simulink model "control2_feedback_linearization"  (R2023b)
settings: Solver=VariableStepAuto  StartTime=0.0  StopTime=20  RelTol=1e-3
values from neighbouring files (symbols this model uses):
  d = obs_r+threshold    (= 0.3)    [main.m]
  initial_position = [0,r]    [main.m]
  obs_r = 0.1    [main.m]
  obs_x = [20]    [main.m]
  obs_y = [20]    [main.m]
  parking_position = [0,0]    [main.m]
  r = 1    [main.m]
  T = 2*pi    (= 6.28318530718)    [main.m]
  t_values = 0:dt:T*1.1    [main.m]
  threshold = 0.2    [main.m]
undefined symbols (not defined in the file or in its folder): params
(part 3 of 3)

== matlab function control2_feedback_linearization/One circle detection/one circle detection ==
  data: t input; x input; regulation_flag output; y input; initial_position input; regulation_flag_previous input; constant input
function regulation_flag  = fcn( t, x,y,initial_position, regulation_flag_previous, constant)
if(regulation_flag_previous==0)
    if (abs(initial_position(1)- x)<0.001 && abs(initial_position(2)-y)<0.001 &&(t>constant))
        regulation_flag=1;
    else 
        regulation_flag=0;
    end
else
    regulation_flag =1;
end

== matlab function control2_feedback_linearization/Trajectory generator/Trajectory generator and obstacle detection3/Subsystem1/Whole trajectory calculation + flatness ==
  data: r input; trajectory_x output; t_values input; T input; trajectory_y output; v_d_array output; omega_d_array output; theta_d_array output; recalculate output; recalculate_obs input; d input; blending input; theta11 input; xd input; yd input; recalculate_obs1 output; old_trajectory_x input; old_trajectory_y input
function [trajectory_x, trajectory_y, v_d_array, omega_d_array, theta_d_array, recalculate,recalculate_obs1]  = fcn( r, t_values,T, recalculate_obs,d, blending, theta11, xd, yd,old_trajectory_x, old_trajectory_y)
    if(~recalculate_obs)
        trajectory_x = zeros(length(t_values), 1);
        trajectory_y = ones(length(t_values), 1);
        % Triangle parameters
        W = 4;  % Base width
        H = 3;  % Height
        x0 = 0;  % Starting x-coordinate
        y0 = 1;  % Starting y-coordinate

        for i = 1:length(t_values)
            t = t_values(i);
            
            if t < T/3
                % Move up diagonally (first leg)
                trajectory_x(i) = x0 + (W/2) * (t / (T/3));
                trajectory_y(i) = y0 + H * (t / (T/3));
                
            elseif t < 2*T/3
                % Move down diagonally (second leg)
                trajectory_x(i) = x0 + (W/2) + (W/2) * ((t - T/3) / (T/3));
                trajectory_y(i) = y0 + H - H * ((t - T/3) / (T/3));
                
            elseif t<T
                % Move horizontally back to start (third leg)
                trajectory_x(i) = x0 + W - W * ((t - 2*T/3) / (T/3));
                trajectory_y(i) = y0;
            else
                trajectory_x(i) = x0;
                trajectory_y(i) = y0;
            end
        end

    else
        % Obstacle was detected: in the point x, y with angle theta
        W = 4;  % Base width
        H = 3;  % Height
        x0 = 0;  % Starting x-coordinate
        y0 = 1;  % Starting y-coordinate
        center_trajectory = [x0+W/2, y0+H/2];
        % Loading previous version of the trajectory 
        % to avoid additional and useless computations of
        % previous desired path
        trajectory_x = old_trajectory_x;
        trajectory_y = old_trajectory_y;
        x1 = xd;
        y1 = yd;
        points = [trajectory_x,trajectory_y];
        [~, start_idx] = min(vecnorm(points - [x1,y1], 2, 2));

        theta1 = -theta11+pi/2;  % Adjusting the angle to get the anglefrom vertical axis (theta11 is wrt horisontal axis)

        % Estimate the obstacle location
        theta_range = linspace(theta1 - pi/4, theta1 + pi/4, 300);
        x_arc = x1 + d * sin(theta_range);
        y_arc = y1 + d * cos(theta_range);



        % Loop through the trajectory points to check for intersections

        obs_x = x1;
        obs_y = y1;
        obs_idx = start_idx;
        for i = start_idx:length(trajectory_x) - 1
            x_traj_seg = [trajectory_x(i), trajectory_x(i + 1)];
            y_traj_seg = [trajectory_y(i), trajectory_y(i + 1)];
            
            for j = 1:length(x_arc) - 1
                x_arc_seg = [x_arc(j), x_arc(j + 1)];
                y_arc_seg = [y_arc(j), y_arc(j + 1)];
                
                % Check if the two segments intersect
                [intersects, ix, iy] = segmentIntersection(x_traj_seg, y_traj_seg, x_arc_seg, y_arc_seg);
        
                if intersects
                    % Intersection found, assign coordinates
                    obs_x = ix;
                    obs_y = iy;
                    obs_idx = i;
                    break; % Exit the loop once intersection is found
                end
             end
            if obs_x ~= x1
                break; 
            end
        end

        % -- > Finding the point where the obstacle avoidance trajectory should 
        % be finished, point from which the robot should continue on
        % the regular trajectory.Creating a circle of radius d, with the 
        % center in [center_obs_x, center_obs_y].
        % After that, finding an intersection of that circle with the 
        % previous trajectory.
    
        theta_values = linspace(0, 2*pi, 500);
        x_circle = obs_x + d * cos(theta_values);
        y_circle = obs_y + d * sin(theta_values);

        % Loop through the trajectory points to check for intersections

        x2 = x1;
        y2 = y1;
        end_idx_trajectory = obs_idx;
        end_idx_circle = 1;

        for i = obs_idx:length(trajectory_x) - 1
            x_traj_seg = [trajectory_x(i), trajectory_x(i + 1)];
            y_traj_seg = [trajectory_y(i), trajectory_y(i + 1)];
            
            for j = 1:length(x_circle) - 1
                x_circle_seg = [x_circle(j), x_circle(j + 1)];
                y_circle_seg = [y_circle(j), y_circle(j + 1)];
                
                % Check if the two segments intersect
                [intersects, ix, iy] = segmentIntersection(x_traj_seg, y_traj_seg, x_circle_seg, y_circle_seg);
        
                if intersects
                    % Intersection found, assign coordinates
                    x2 = ix;
                    y2 = iy;
                    end_idx_trajectory = i;
                    end_idx_circle = j;
                    break; 
                end
            end
            if x2 ~= x1, break; end
        end

        % --> Finding the longer arc of the circle around obstacle
        % This will be the desired obstacle avoidance path
        points = [x_circle' y_circle']; % Nx2 array
        [~, idx1] = min(vecnorm(points - [x1,y1], 2, 2));
        idx2 = end_idx_circle;
        
        if idx1 < idx2
            arc1 = points(idx1:idx2, :);       
            arc2 = [points(idx2:end, :); points(1:idx1, :)];
        else
            arc1 = points(idx2:idx1, :);       
            arc2 = [points(idx1:end, :); points(1:idx2, :)];
        end
        
        idx_point1 = floor(size(arc1,1)/2);
        idx_point2 = floor(size(arc2,1)/2);
        
        distance1 = (arc1(idx_point1,1)-center_trajectory(1))^2+(arc1(idx_point1,2)-center_trajectory(2))^2;
        distance2 =  (arc2(idx_point2,1)-center_trajectory(1))^2+(arc2(idx_point2,2)-center_trajectory(2))^2;
        
        if distance1>distance2
            longer_arc = arc1;
        else
            longer_arc = arc2;
        end
        % Reverse if needed
        if(abs(longer_arc(1,1)-x1)>abs(longer_arc(1,1)-x2))
            longer_arc = flip(longer_arc);
        end


        % --> Creating a new trajectory
        idx1 = start_idx;
        idx2 = end_idx_trajectory;
        % Change of the trajectory is allowed if the ordering is okay
        % first indexwise is the point of detection and then the obstacle
        % (should always be satisfied)
        if(idx1<idx2 && t_values(idx2)<T)

            n_points = idx2 - idx1 + 1;
            total_points = size(longer_arc,1);
            indices = round(linspace(1, total_points, n_points));
            % Smoothly blend the two trajectories if needed
            trajectory_avoid_x = longer_arc(indices,1);
            trajectory_avoid_y = longer_arc(indices,2);
            trajectory_old_x = trajectory_x(idx1:idx2);
            trajectory_old_y = trajectory_y(idx1:idx2);

            trajectory_x(idx1:idx2) = blending*trajectory_avoid_x + (1-blending)*trajectory_old_x;
            trajectory_y(idx1:idx2) = blending*trajectory_avoid_y + (1-blending)*trajectory_old_y;

        end
    end

    recalculate_obs1 = 0;
    recalculate = 0;


    dt = t_values(2) - t_values(1);

    %  Derivatives
    dx_d = gradient(trajectory_x, dt);
    dy_d = gradient(trajectory_y, dt);
    ddx_d = gradient(dx_d, dt);
    ddy_d = gradient(dy_d, dt);
    
    v_d_array = sqrt(dx_d.^2 + dy_d.^2);
    omega_d_array = (ddy_d .* dx_d - ddx_d .* dy_d) ./ ((dx_d.^2 + dy_d.^2)+eps);
    theta_d_array=atan2(dy_d,dx_d);

end

== matlab function control2_feedback_linearization/Trajectory generator/Trajectory generator and obstacle detection3/Subsystem3/Triggered Subsystem/MATLAB Function1 ==
  data: t input; t_values input; trajectory_x input; x_d output; trajectory_y input; y_d output; v_d output; omega_d output; theta_d output; v_d_array input; omega_d_array input; theta_d_array input; i input; new_i output
function [x_d, y_d, v_d, omega_d, theta_d, new_i] = fcn(t, t_values, trajectory_x, trajectory_y, v_d_array, omega_d_array, theta_d_array,i)

    % When the block is not enabled (on the start),this is used to give initial position
    if (i==0)
        new_i=1;
    else
        new_i =i;
    end

    [~, idx] = min(abs(t_values - t));  % closest index to current time
    if(t>t_values(end))
        idx = length(t_values);
    end
    % Position
    x_d = trajectory_x(idx);  
    y_d = trajectory_y(idx);

    % Flatness
    v_d = v_d_array(idx);  
    omega_d = omega_d_array(idx);
    theta_d = theta_d_array(idx);

== matlab function control2_feedback_linearization/Regulation task: controller and model /Controller with polar coordinates/Transformation to Cartesian coordinates ==
  data: x output; rho input; y output; gamma input; delta input; theta output
function [x, y, theta] = fcn(rho, gamma, delta)
gamma1 = wrapToPi(gamma);
delta1 = wrapToPi(delta);

theta = delta1 - gamma1; 

x = -rho*cos(delta1);
y = -rho*sin(delta1);

== matlab function control2_feedback_linearization/Regulation task: controller and model /Controller with polar coordinates/Transformation to polar coordinates ==
  data: rho output; x input; gamma output; y input; theta input; delta output
function [rho, gamma, delta] = fcn(x, y, theta)

rho = sqrt(x^2+y^2);
gamma = wrapToPi(atan2(y, x) - theta + pi);
delta = wrapToPi(gamma + theta);

== matlab function control2_feedback_linearization/Regulation task: controller and model /Controller with polar coordinates/Unicycle model: polar coordinates ==
  data: rho input; gamma input; u input; rho_dot output; omega input; gamma_dot output; delta_dot output; regulation_flag input
function [rho_dot, gamma_dot, delta_dot] = model(rho, gamma, u, omega, regulation_flag)
if(regulation_flag)
    rho_dot = -u*rho*cos(gamma);
    gamma_dot = sin(gamma)*u-omega;
    delta_dot = sin(gamma)*u;
else
    rho_dot = 0;
    gamma_dot = 0;
    delta_dot = 0;
end

== matlab function control2_feedback_linearization/Regulation task: controller and model /Regulation controller choice ==
  data: x1 input; y1 input; theta1 input; controller_choice input; x_out output; x2 input; y2 input; theta2 input; y_out output; theta_out output
function [x_out, y_out, theta_out] = fcn(x1, y1, theta1, controller_choice, x2, y2, theta2 )
if(controller_choice==1)
    x_out = x1;
    y_out = y1;
    theta_out = theta1;
else
    x_out = x2;
    y_out = y2;
    theta_out = theta2;
end

== matlab function control2_feedback_linearization/Second controller: with b1/MATLAB Function1 ==
  data: u1 input; u2 input; b input; theta input; v output; omega output
function [v,omega] = T_inverse(u1,u2,b,theta)
T=[cos(theta),-b*sin(theta);
    sin(theta),b*cos(theta)];
%instead of explicitly calculating the inverse of using inv(T), 
% using matrix division (\) is numerically more stable.
    velocities = T \ [u1; u2];
    
    % Extract linear and angular velocities
    v = velocities(1);
    omega = velocities(2);
end

== matlab function control2_feedback_linearization/Second controller: with b1/MATLAB Function2 ==
  data: x_d input; xb_d output; y_d input; yb_d output; b input; theta_d input
function [xb_d,yb_d] = P2B(x_d,y_d,b, theta_d)
xb_d=x_d+b*cos(theta_d);
yb_d=y_d+b*sin(theta_d);
end

== matlab function control2_feedback_linearization/Second controller: with b1/MATLAB Function3 ==
  data: eb_x input; eb_y input; u1i output; u2i output; kp1 input; kp2 input
function [u1i,u2i]=error(eb_x, eb_y,kp1,kp2)
u1i=kp1*eb_x;
u2i=kp2*eb_y;
end

== matlab function control2_feedback_linearization/Trajectory generator/Trajectory generator and obstacle detection/MATLAB Function ==
  data: initial_position input; x1 input; y1 input; v1 input; omega1 input; theta1 input; i input; x output; y output; v output; omega output; theta output
function [x,y,v,omega,theta] = fcn(initial_position, x1,y1,v1, omega1, theta1,i)

if(i == 0)
    x = initial_position(1);
    y = initial_position(2);
    v = 0;
    omega = 0;
    theta=0;
else
    x = x1;
    y = y1;
    v = v1;
    omega = omega1;
    theta=theta1;
end
